simulink model "HexWaRo"  (R2012b)
settings: Solver=ode45  StartTime=0.0  StopTime=2  RelTol=1e-3
libraries: mblibv1 x79
(part 2 of 2)

== system HexWaRo/Subsystem3/Contact Force ==
  Body Actuator : mblibv1/Sensors &  Actuators/Body Actuator  UpdateFromCAD=off  PhysicalDomain=Mechanical  PortType=blob  ActuationStyle=Force  AngleUnits=deg  ArcVelocityUnits=deg/s  ArcAccelerationUnits=deg/s^2  CoordPositionUnits=m  VelocityUnits=m/s  AccelerationUnits=m/s^2  ForceUnits=N  TorqueUnits=N-m  ActiveIO=on  Width=3  DialogClass=MechanicalActuatorBlock  ReferenceFrame=Absolute (INERTIAL)  Angle=off  CoordPosition=on  Force=on  Torque=off
  Body Sensor : mblibv1/Sensors &  Actuators/Body Sensor  UpdateFromCAD=off  PhysicalDomain=Mechanical  PortType=blob  Muxed=off  Pose=off  Angle=on  AngleUnits=deg  ArcVelocity=off  ArcVelocityUnits=deg/s  ArcAcceleration=off  ArcAccelerationUnits=deg/s^2  CoordPosition=on  CoordPositionUnits=m  Velocity=on  VelocityUnits=m/s  Acceleration=off  AccelerationUnits=m/s^2  Quaternion=on  QuaternionDT=off  QuaternionDDT=off  QuaternionUnits=off  OutputVector=[ 3 3 ]  ActiveIO=on  Width=6  DialogClass=MechanicalSensorBlock  ReferenceFrame=Absolute (World)
  Force Law : Subsystem
  Mechanical Branching Bar : mblibv1/Utilities/Mechanical Branching Bar  LConnTagsString=_newl0  RConnTagsString=SA0|SA1  UpdateFromCAD=off  DialogClass=MechanicalBranchingBarBlock  NumSAPorts=2
  CG : PMIOPort  Tag=PMCPort  Port=1  Side=Left
  wires:
  Body Sensor/1 -> Force Law/1(pos)  "Position (m)"
  Body Sensor/2 -> Force Law/2(vel)  "Velocity (m/s)"
  Force Law/1(force) -> Body Actuator/1  "Force (N)"
  connections:
  Mechanical Branching Bar/LConn1 -- CG/RConn1
  Body Actuator/RConn1 -- Mechanical Branching Bar/RConn2
  Body Sensor/LConn1 -- Mechanical Branching Bar/RConn1

== system HexWaRo/Subsystem4/Contact Force ==
  Body Actuator : mblibv1/Sensors &  Actuators/Body Actuator  UpdateFromCAD=off  PhysicalDomain=Mechanical  PortType=blob  ActuationStyle=Force  AngleUnits=deg  ArcVelocityUnits=deg/s  ArcAccelerationUnits=deg/s^2  CoordPositionUnits=m  VelocityUnits=m/s  AccelerationUnits=m/s^2  ForceUnits=N  TorqueUnits=N-m  ActiveIO=on  Width=3  DialogClass=MechanicalActuatorBlock  ReferenceFrame=Absolute (INERTIAL)  Angle=off  CoordPosition=on  Force=on  Torque=off
  Body Sensor : mblibv1/Sensors &  Actuators/Body Sensor  UpdateFromCAD=off  PhysicalDomain=Mechanical  PortType=blob  Muxed=off  Pose=off  Angle=on  AngleUnits=deg  ArcVelocity=off  ArcVelocityUnits=deg/s  ArcAcceleration=off  ArcAccelerationUnits=deg/s^2  CoordPosition=on  CoordPositionUnits=m  Velocity=on  VelocityUnits=m/s  Acceleration=off  AccelerationUnits=m/s^2  Quaternion=on  QuaternionDT=off  QuaternionDDT=off  QuaternionUnits=off  OutputVector=[ 3 3 ]  ActiveIO=on  Width=6  DialogClass=MechanicalSensorBlock  ReferenceFrame=Absolute (World)
  Force Law : Subsystem
  Mechanical Branching Bar : mblibv1/Utilities/Mechanical Branching Bar  LConnTagsString=_newl0  RConnTagsString=SA0|SA1  UpdateFromCAD=off  DialogClass=MechanicalBranchingBarBlock  NumSAPorts=2
  CG : PMIOPort  Tag=PMCPort  Port=1  Side=Left
  wires:
  Force Law/1(force) -> Body Actuator/1  "Force (N)"
  Body Sensor/2 -> Force Law/2(vel)  "Velocity (m/s)"
  Body Sensor/1 -> Force Law/1(pos)  "Position (m)"
  connections:
  Body Sensor/LConn1 -- Mechanical Branching Bar/RConn1
  Body Actuator/RConn1 -- Mechanical Branching Bar/RConn2
  Mechanical Branching Bar/LConn1 -- CG/RConn1

== system HexWaRo/Subsystem5/Contact Force ==
  Body Actuator : mblibv1/Sensors &  Actuators/Body Actuator  UpdateFromCAD=off  PhysicalDomain=Mechanical  PortType=blob  ActuationStyle=Force  AngleUnits=deg  ArcVelocityUnits=deg/s  ArcAccelerationUnits=deg/s^2  CoordPositionUnits=m  VelocityUnits=m/s  AccelerationUnits=m/s^2  ForceUnits=N  TorqueUnits=N-m  ActiveIO=on  Width=3  DialogClass=MechanicalActuatorBlock  ReferenceFrame=Absolute (INERTIAL)  Angle=off  CoordPosition=on  Force=on  Torque=off
  Body Sensor : mblibv1/Sensors &  Actuators/Body Sensor  UpdateFromCAD=off  PhysicalDomain=Mechanical  PortType=blob  Muxed=off  Pose=off  Angle=on  AngleUnits=deg  ArcVelocity=off  ArcVelocityUnits=deg/s  ArcAcceleration=off  ArcAccelerationUnits=deg/s^2  CoordPosition=on  CoordPositionUnits=m  Velocity=on  VelocityUnits=m/s  Acceleration=off  AccelerationUnits=m/s^2  Quaternion=on  QuaternionDT=off  QuaternionDDT=off  QuaternionUnits=off  OutputVector=[ 3 3 ]  ActiveIO=on  Width=6  DialogClass=MechanicalSensorBlock  ReferenceFrame=Absolute (World)
  Force Law : Subsystem
  Mechanical Branching Bar : mblibv1/Utilities/Mechanical Branching Bar  LConnTagsString=_newl0  RConnTagsString=SA0|SA1  UpdateFromCAD=off  DialogClass=MechanicalBranchingBarBlock  NumSAPorts=2
  CG : PMIOPort  Tag=PMCPort  Port=1  Side=Left
  wires:
  Body Sensor/1 -> Force Law/1(pos)  "Position (m)"
  Body Sensor/2 -> Force Law/2(vel)  "Velocity (m/s)"
  Force Law/1(force) -> Body Actuator/1  "Force (N)"
  connections:
  Mechanical Branching Bar/LConn1 -- CG/RConn1
  Body Actuator/RConn1 -- Mechanical Branching Bar/RConn2
  Body Sensor/LConn1 -- Mechanical Branching Bar/RConn1

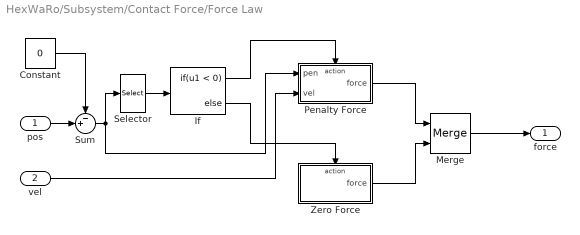
== system HexWaRo/Subsystem/Contact Force/Force Law ==
  pos : Inport
  vel : Inport  Port=2
  Constant : Constant  Value=0
  If : If  IfExpression=u1 < 0
  Merge : Merge  InitialOutput=0  InputPortOffsets=0
  Penalty Force : Subsystem  TreatAsAtomicUnit=on
  Selector : Selector  InputPortWidth=3  IndexOptions=Index vector (dialog)  Indices=[3]  OutputSizes=1
  Sum : Sum  Inputs=-+|  SaturateOnIntegerOverflow=on
  Zero Force : Subsystem  TreatAsAtomicUnit=on
  force : Outport
  wires:
  Selector/1 -> If/1
  If/1 -> Penalty Force/Action
  Merge/1 -> force/1
  Zero Force/1(force) -> Merge/2
  Penalty Force/1(force) -> Merge/1
  If/2 -> Zero Force/Action
  vel/1 -> Penalty Force/2(vel)
  Constant/1 -> Sum/1
  Sum/1 -> Penalty Force/1(pen), Selector/1
  pos/1 -> Sum/2

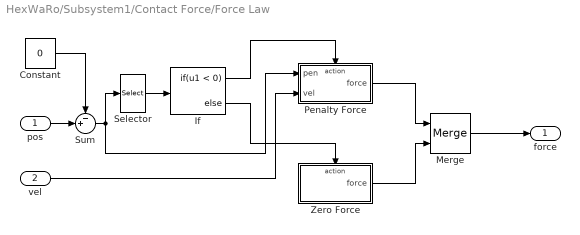
== system HexWaRo/Subsystem1/Contact Force/Force Law ==
  pos : Inport
  vel : Inport  Port=2
  Constant : Constant  Value=0
  If : If  IfExpression=u1 < 0
  Merge : Merge  InitialOutput=0  InputPortOffsets=0
  Penalty Force : Subsystem  TreatAsAtomicUnit=on
  Selector : Selector  InputPortWidth=3  IndexOptions=Index vector (dialog)  Indices=[3]  OutputSizes=1
  Sum : Sum  Inputs=-+|  SaturateOnIntegerOverflow=on
  Zero Force : Subsystem  TreatAsAtomicUnit=on
  force : Outport
  wires:
  pos/1 -> Sum/2
  Sum/1 -> Selector/1, Penalty Force/1(pen)
  Constant/1 -> Sum/1
  vel/1 -> Penalty Force/2(vel)
  If/2 -> Zero Force/Action
  Penalty Force/1(force) -> Merge/1
  Zero Force/1(force) -> Merge/2
  Merge/1 -> force/1
  If/1 -> Penalty Force/Action
  Selector/1 -> If/1

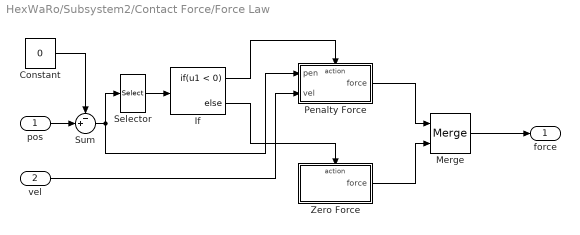
== system HexWaRo/Subsystem2/Contact Force/Force Law ==
  pos : Inport
  vel : Inport  Port=2
  Constant : Constant  Value=0
  If : If  IfExpression=u1 < 0
  Merge : Merge  InitialOutput=0  InputPortOffsets=0
  Penalty Force : Subsystem  TreatAsAtomicUnit=on
  Selector : Selector  InputPortWidth=3  IndexOptions=Index vector (dialog)  Indices=[3]  OutputSizes=1
  Sum : Sum  Inputs=-+|  SaturateOnIntegerOverflow=on
  Zero Force : Subsystem  TreatAsAtomicUnit=on
  force : Outport
  wires:
  Selector/1 -> If/1
  If/1 -> Penalty Force/Action
  Merge/1 -> force/1
  Zero Force/1(force) -> Merge/2
  Penalty Force/1(force) -> Merge/1
  If/2 -> Zero Force/Action
  vel/1 -> Penalty Force/2(vel)
  Constant/1 -> Sum/1
  Sum/1 -> Penalty Force/1(pen), Selector/1
  pos/1 -> Sum/2

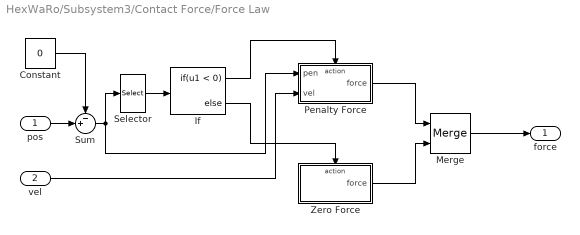
== system HexWaRo/Subsystem3/Contact Force/Force Law ==
  pos : Inport
  vel : Inport  Port=2
  Constant : Constant  Value=0
  If : If  IfExpression=u1 < 0
  Merge : Merge  InitialOutput=0  InputPortOffsets=0
  Penalty Force : Subsystem  TreatAsAtomicUnit=on
  Selector : Selector  InputPortWidth=3  IndexOptions=Index vector (dialog)  Indices=[3]  OutputSizes=1
  Sum : Sum  Inputs=-+|  SaturateOnIntegerOverflow=on
  Zero Force : Subsystem  TreatAsAtomicUnit=on
  force : Outport
  wires:
  pos/1 -> Sum/2
  Sum/1 -> Selector/1, Penalty Force/1(pen)
  Constant/1 -> Sum/1
  vel/1 -> Penalty Force/2(vel)
  If/2 -> Zero Force/Action
  Penalty Force/1(force) -> Merge/1
  Zero Force/1(force) -> Merge/2
  Merge/1 -> force/1
  If/1 -> Penalty Force/Action
  Selector/1 -> If/1

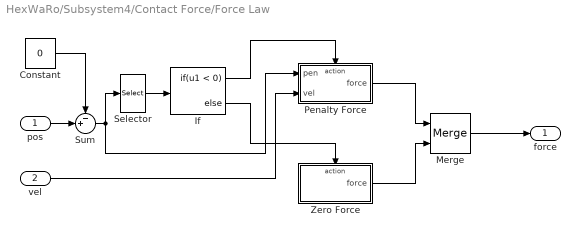
== system HexWaRo/Subsystem4/Contact Force/Force Law ==
  pos : Inport
  vel : Inport  Port=2
  Constant : Constant  Value=0
  If : If  IfExpression=u1 < 0
  Merge : Merge  InitialOutput=0  InputPortOffsets=0
  Penalty Force : Subsystem  TreatAsAtomicUnit=on
  Selector : Selector  InputPortWidth=3  IndexOptions=Index vector (dialog)  Indices=[3]  OutputSizes=1
  Sum : Sum  Inputs=-+|  SaturateOnIntegerOverflow=on
  Zero Force : Subsystem  TreatAsAtomicUnit=on
  force : Outport
  wires:
  Selector/1 -> If/1
  If/1 -> Penalty Force/Action
  Merge/1 -> force/1
  Zero Force/1(force) -> Merge/2
  Penalty Force/1(force) -> Merge/1
  If/2 -> Zero Force/Action
  vel/1 -> Penalty Force/2(vel)
  Constant/1 -> Sum/1
  Sum/1 -> Penalty Force/1(pen), Selector/1
  pos/1 -> Sum/2

== system HexWaRo/Subsystem5/Contact Force/Force Law ==
  pos : Inport
  vel : Inport  Port=2
  Constant : Constant  Value=0
  If : If  IfExpression=u1 < 0
  Merge : Merge  InitialOutput=0  InputPortOffsets=0
  Penalty Force : Subsystem  TreatAsAtomicUnit=on
  Selector : Selector  InputPortWidth=3  IndexOptions=Index vector (dialog)  Indices=[3]  OutputSizes=1
  Sum : Sum  Inputs=-+|  SaturateOnIntegerOverflow=on
  Zero Force : Subsystem  TreatAsAtomicUnit=on
  force : Outport
  wires:
  pos/1 -> Sum/2
  Sum/1 -> Selector/1, Penalty Force/1(pen)
  Constant/1 -> Sum/1
  vel/1 -> Penalty Force/2(vel)
  If/2 -> Zero Force/Action
  Penalty Force/1(force) -> Merge/1
  Zero Force/1(force) -> Merge/2
  Merge/1 -> force/1
  If/1 -> Penalty Force/Action
  Selector/1 -> If/1

== system HexWaRo/Subsystem/Contact Force/Force Law/Penalty Force ==
  pen : Inport
  vel : Inport  Port=2
  Action Port : ActionPort  ActionType=then
  Gain : Gain  Gain=[0 0 0;0 0 0;0 0 -1500]  Multiplication=Matrix(K*u)  SaturateOnIntegerOverflow=on  OutDataTypeStr=Inherit: Same as input  ParamDataTypeStr=Inherit: Same as input
  Gain1 : Gain  Gain=[0 0 0;0 0 0;0 0 -50]  Multiplication=Matrix(K*u)  SaturateOnIntegerOverflow=on  OutDataTypeStr=Inherit: Same as input  ParamDataTypeStr=Inherit: Same as input
  Saturation : Saturate  UpperLimit=inf  LowerLimit=0
  Sum : Sum  Inputs=|++  SaturateOnIntegerOverflow=on
  force : Outport  InitialOutput=0
  wires:
  Saturation/1 -> force/1
  vel/1 -> Gain1/1
  Gain1/1 -> Sum/2
  Sum/1 -> Saturation/1
  Gain/1 -> Sum/1
  pen/1 -> Gain/1

== system HexWaRo/Subsystem/Contact Force/Force Law/Zero Force ==
  Action Port : ActionPort  ActionType=else
  Zero Force : Constant  Value=[0;0;0]
  force : Outport  InitialOutput=0
  wires:
  Zero Force/1 -> force/1

== system HexWaRo/Subsystem1/Contact Force/Force Law/Penalty Force ==
  pen : Inport
  vel : Inport  Port=2
  Action Port : ActionPort  ActionType=then
  Gain : Gain  Gain=[0 0 0;0 0 0;0 0 -1500]  Multiplication=Matrix(K*u)  SaturateOnIntegerOverflow=on  OutDataTypeStr=Inherit: Same as input  ParamDataTypeStr=Inherit: Same as input
  Gain1 : Gain  Gain=[0 0 0;0 0 0;0 0 -50]  Multiplication=Matrix(K*u)  SaturateOnIntegerOverflow=on  OutDataTypeStr=Inherit: Same as input  ParamDataTypeStr=Inherit: Same as input
  Saturation : Saturate  UpperLimit=inf  LowerLimit=0
  Sum : Sum  Inputs=|++  SaturateOnIntegerOverflow=on
  force : Outport  InitialOutput=0
  wires:
  pen/1 -> Gain/1
  Gain/1 -> Sum/1
  Sum/1 -> Saturation/1
  Gain1/1 -> Sum/2
  vel/1 -> Gain1/1
  Saturation/1 -> force/1

== system HexWaRo/Subsystem1/Contact Force/Force Law/Zero Force ==
  Action Port : ActionPort  ActionType=else
  Zero Force : Constant  Value=[0;0;0]
  force : Outport  InitialOutput=0
  wires:
  Zero Force/1 -> force/1

== system HexWaRo/Subsystem2/Contact Force/Force Law/Penalty Force ==
  pen : Inport
  vel : Inport  Port=2
  Action Port : ActionPort  ActionType=then
  Gain : Gain  Gain=[0 0 0;0 0 0;0 0 -1500]  Multiplication=Matrix(K*u)  SaturateOnIntegerOverflow=on  OutDataTypeStr=Inherit: Same as input  ParamDataTypeStr=Inherit: Same as input
  Gain1 : Gain  Gain=[0 0 0;0 0 0;0 0 -50]  Multiplication=Matrix(K*u)  SaturateOnIntegerOverflow=on  OutDataTypeStr=Inherit: Same as input  ParamDataTypeStr=Inherit: Same as input
  Saturation : Saturate  UpperLimit=inf  LowerLimit=0
  Sum : Sum  Inputs=|++  SaturateOnIntegerOverflow=on
  force : Outport  InitialOutput=0
  wires:
  Saturation/1 -> force/1
  vel/1 -> Gain1/1
  Gain1/1 -> Sum/2
  Sum/1 -> Saturation/1
  Gain/1 -> Sum/1
  pen/1 -> Gain/1

== system HexWaRo/Subsystem2/Contact Force/Force Law/Zero Force ==
  Action Port : ActionPort  ActionType=else
  Zero Force : Constant  Value=[0;0;0]
  force : Outport  InitialOutput=0
  wires:
  Zero Force/1 -> force/1

== system HexWaRo/Subsystem3/Contact Force/Force Law/Penalty Force ==
  pen : Inport
  vel : Inport  Port=2
  Action Port : ActionPort  ActionType=then
  Gain : Gain  Gain=[0 0 0;0 0 0;0 0 -1500]  Multiplication=Matrix(K*u)  SaturateOnIntegerOverflow=on  OutDataTypeStr=Inherit: Same as input  ParamDataTypeStr=Inherit: Same as input
  Gain1 : Gain  Gain=[0 0 0;0 0 0;0 0 -50]  Multiplication=Matrix(K*u)  SaturateOnIntegerOverflow=on  OutDataTypeStr=Inherit: Same as input  ParamDataTypeStr=Inherit: Same as input
  Saturation : Saturate  UpperLimit=inf  LowerLimit=0
  Sum : Sum  Inputs=|++  SaturateOnIntegerOverflow=on
  force : Outport  InitialOutput=0
  wires:
  pen/1 -> Gain/1
  Gain/1 -> Sum/1
  Sum/1 -> Saturation/1
  Gain1/1 -> Sum/2
  vel/1 -> Gain1/1
  Saturation/1 -> force/1

== system HexWaRo/Subsystem3/Contact Force/Force Law/Zero Force ==
  Action Port : ActionPort  ActionType=else
  Zero Force : Constant  Value=[0;0;0]
  force : Outport  InitialOutput=0
  wires:
  Zero Force/1 -> force/1

== system HexWaRo/Subsystem4/Contact Force/Force Law/Penalty Force ==
  pen : Inport
  vel : Inport  Port=2
  Action Port : ActionPort  ActionType=then
  Gain : Gain  Gain=[0 0 0;0 0 0;0 0 -1500]  Multiplication=Matrix(K*u)  SaturateOnIntegerOverflow=on  OutDataTypeStr=Inherit: Same as input  ParamDataTypeStr=Inherit: Same as input
  Gain1 : Gain  Gain=[0 0 0;0 0 0;0 0 -50]  Multiplication=Matrix(K*u)  SaturateOnIntegerOverflow=on  OutDataTypeStr=Inherit: Same as input  ParamDataTypeStr=Inherit: Same as input
  Saturation : Saturate  UpperLimit=inf  LowerLimit=0
  Sum : Sum  Inputs=|++  SaturateOnIntegerOverflow=on
  force : Outport  InitialOutput=0
  wires:
  Saturation/1 -> force/1
  vel/1 -> Gain1/1
  Gain1/1 -> Sum/2
  Sum/1 -> Saturation/1
  Gain/1 -> Sum/1
  pen/1 -> Gain/1

== system HexWaRo/Subsystem4/Contact Force/Force Law/Zero Force ==
  Action Port : ActionPort  ActionType=else
  Zero Force : Constant  Value=[0;0;0]
  force : Outport  InitialOutput=0
  wires:
  Zero Force/1 -> force/1

== system HexWaRo/Subsystem5/Contact Force/Force Law/Penalty Force ==
  pen : Inport
  vel : Inport  Port=2
  Action Port : ActionPort  ActionType=then
  Gain : Gain  Gain=[0 0 0;0 0 0;0 0 -1500]  Multiplication=Matrix(K*u)  SaturateOnIntegerOverflow=on  OutDataTypeStr=Inherit: Same as input  ParamDataTypeStr=Inherit: Same as input
  Gain1 : Gain  Gain=[0 0 0;0 0 0;0 0 -50]  Multiplication=Matrix(K*u)  SaturateOnIntegerOverflow=on  OutDataTypeStr=Inherit: Same as input  ParamDataTypeStr=Inherit: Same as input
  Saturation : Saturate  UpperLimit=inf  LowerLimit=0
  Sum : Sum  Inputs=|++  SaturateOnIntegerOverflow=on
  force : Outport  InitialOutput=0
  wires:
  pen/1 -> Gain/1
  Gain/1 -> Sum/1
  Sum/1 -> Saturation/1
  Gain1/1 -> Sum/2
  vel/1 -> Gain1/1
  Saturation/1 -> force/1

== system HexWaRo/Subsystem5/Contact Force/Force Law/Zero Force ==
  Action Port : ActionPort  ActionType=else
  Zero Force : Constant  Value=[0;0;0]
  force : Outport  InitialOutput=0
  wires:
  Zero Force/1 -> force/1

== matlab function HexWaRo/MATLAB Function ==
  data: OP input; ta1 output; roll input; pitch input; yaw input; ta2 output; ta3 output; ta4 output; ta5 output; ta6 output; exitflag output
function [ta1,ta2,ta3,ta4,ta5,ta6,exitflag] = fcn(OP,roll,pitch,yaw)
%#codegen

% THIS PROGRAM IS GOING TO TAKE ALL THE GROUND COORDINATES TO MOVING
% PLATFORM FRAME AND CALCULATE INVERSE KINEMATIC THERE.
% ADVANCED ROBOTIC PROJECT - Supervisor Dr Osguie
%  - Shahriari Summer 2012

%% INITIALIZING THE PROBLEM ==============================
l0=2.5;%cm
l1=7.4;%cm
l2=11.4;%cm
lc=l0;
lf=l1;
lt=l2;
global l0 l1 l2 lt lf lc 
P=zeros(3,1);
h=7.87; % Radios of platform
P1=P+[h*sin(pi/6);h*cos(pi/6);0];
P2=P+[h;0;0];
P3=P+[h*sin(pi/6);-h*cos(pi/6);0];
P4=P+[-h*sin(pi/6);-h*cos(pi/6);0];
P5=P+[-h;0;0];
P6=P+[-h*sin(pi/6);h*cos(pi/6);0];
P_MB=[P1,P2,P3,P4,P5,P6];% The edges of the body where limbs begin in main bodie's frame/
P_MB=P_MB([2,1,3],:);
% Giving a sample legs tips position:
Q1=[7.5000;12.9904;0];
phi=[0,pi/3,2*pi/3,pi,4*pi/3,5*pi/3];
for i=1:6
Q2(:,i)=(rot(phi(i))*Q1);
end
Q2=Q2([2,1,3],:);
%% Configuration =========================================================
% OP=[0;0;6]; % the position of the frame of main body from ground frame.
Ltip=Q2;
% yaw=0;% Around Z
% roll=0;% Around X
% pitch=0;% Around Y
%% Define Legs tip in Main body frame====================================

Trn_op=TrnoPe(yaw,pitch,roll,-OP);
for i=1:6
    Ltip_MB(:,i)=Trn_op*[Ltip(:,i);1];
end
Ltip_MB=Ltip_MB(1:3,:);

%% solving inverse Kinematic Problem===========================
% first we should define the X,Y,Z distance of the leg tip from the leg
% frame positioned on the body ( P1,P2...)

Ltip_JF=Ltip_MB-P_MB; % Leg tip in Joint Frame
% global Ltip_JF
% [t,fval,exitflag]=fsolve('Legs',zeros(3,6));
for i=1:6    
    x=Ltip_JF(1,i);
    y=Ltip_JF(2,i);
    z=Ltip_JF(3,i);
       
        t1(i)=atan2(y,x);
        c=((x-l0*cos(t1(i)))^2+(y-l0*sin(t1(i)))^2+z^2)^.5;
        B=acos((-l2^2+l1^2+c^2)/(2*l1*c));
        t2(i)=(asin(-z/c)-B);
        C1=pi/2-B;
        h=l1*sin(B);
        C2=acos(h/l2);
        t3(i)=(pi-C1-C2);
          
end
ExFl=imag(t1)+imag(t2)+imag(t3);
ExFl=mean(ExFl);
if ExFl==0
exitflag=1;
else
    exitflag=-1;
end
ta1=[t1(1),t2(1),t3(1)]';
ta2=[t1(2),t2(2),t3(2)]';
ta3=[t1(3),t2(3),t3(3)]';
ta4=[t1(4),t2(4),t3(4)]';
ta5=[t1(5),t2(5),t3(5)]';
ta6=[t1(6),t2(6),t3(6)]';
